simulink model "myproject_task"  (Simulink 3.00)
libraries: genlib x4, mathlib x3, arclib x1

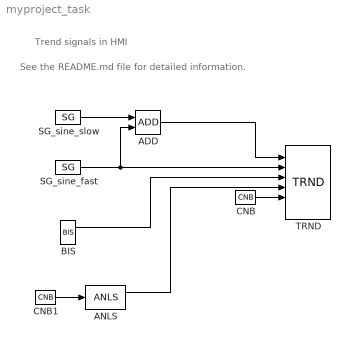
== system myproject_task ==
  note: See the README.md file for detailed information.
  note: Trend signals in HMI
  ADD : mathlib/ADD
  ANLS : genlib/ANLS  y0=5  t1=5  y1=10  t2=7  y2=10  t3=7  y3=8  t4=10  y4=8  RPT=on
  BIS : genlib/BIS  Y0=off  t1=0.2  t2=0.4  t3=0.6  t4=0.8  t5=2  t6=3  t7=6  t8=10  RPT=on
  CNB : mathlib/CNB  YCN=on
  CNB1 : mathlib/CNB  YCN=on
  SG_sine_fast : genlib/SG  isig=1: SINE  amp=3  freq=0.09  phase=0  ifrunit=1: Hz  iphunit=1: degrees  offset=-4
  SG_sine_slow : genlib/SG  isig=1: SINE  amp=10  freq=0.025  phase=0  ifrunit=1: Hz  iphunit=1: degrees  offset=20
  TRND : arclib/TRND  n=4  l=600  btype=8: Double  ptype1=1: Store  ptype2=1: Store  ptype3=1: Store  ptype4=1: Store  pfac=1  afac=0  arc=0  id=1  Title=Signal generators demo  timesrc=1: CORETIMER
  wires:
  ADD/1 -> TRND/1
  ANLS/1 -> TRND/4
  BIS/1 -> TRND/3
  CNB/1 -> TRND/5
  CNB1/1 -> ANLS/1
  SG_sine_fast/1 -> ADD/2, TRND/2
  SG_sine_slow/1 -> ADD/1
